simulink model "radar_sensitivity"  (R2016b)
settings: Solver=VariableStepAuto  StartTime=0.0  StopTime=50  RelTol=1e-3
values from neighbouring files (symbols this model uses):
  K = gain(x)    [radar_sweep.m]    (also in sweep.m; sweep_1.m; sweep_2.m; wind_sweep.m)
settings Model: Creator=ammar_laptop  LastModifiedBy=ammar_laptop

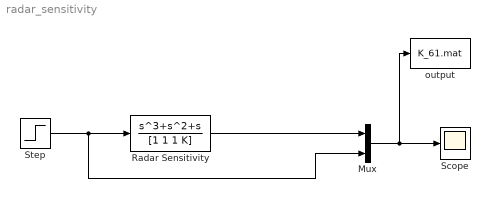
== system radar_sensitivity ==
  Mux : Mux  Inputs=2
  Radar Sensitivity : TransferFcn  Numerator=[1 1 1 0]  Denominator=[1 1 1 K]
  Scope : Scope
  Step : Step  SampleTime=0
  output : ToFile  Filename=K_61.mat  SaveFormat=Timeseries
  wires:
  Step/1 -> Mux/2, Radar Sensitivity/1
  Radar Sensitivity/1 -> Mux/1
  Mux/1 -> output/1, Scope/1
